simulink model "pidACCsystem"  (R2022a)
settings: Solver=FixedStepAuto  StartTime=0.0  StopTime=T  RelTol=1e-3
values from neighbouring files (symbols this model uses):
  t_gap = 1.4    [PreRun.m]
  Ts = 1e-2    (= 0.01)    [PreRun.m]
  v0_ego_1 = 20/9    (= 2.22222222222)    [PreRun.m]
  v0_ego_2 = 20/9    (= 2.22222222222)    [PreRun.m]
  v0_ego_3 = 20/9    (= 2.22222222222)    [PreRun.m]
  v0_lead = 25/9    (= 2.77777777778)    [PreRun.m]
  x0_ego_1 = x0_lead - (10 + t_gap*v0_ego_1)    (= 56.8888888889)    [PreRun.m]
  x0_ego_2 = x0_ego_1 - (10 + t_gap*v0_ego_2)    (= 43.7777777778)    [PreRun.m]
  x0_ego_3 = x0_ego_2 - (10 + t_gap*v0_ego_3)    (= 30.6666666667)    [PreRun.m]
  x0_lead = 70    [PreRun.m]
libraries: eeStairGenerator x1
settings Model: Creator=The MathWorks, Inc.  LastModifiedBy=SAMEER TALWAR
settings SolverCC: AlgebraicLoopSolver=TrustRegion
settings DataIOCC: ReturnWorkspaceOutputs=off
settings DebuggingCC: UnconnectedInputMsg=warning  UnconnectedOutputMsg=warning  UnconnectedLineMsg=warning  SFMachineParentedDataDiag=warning  ArithmeticOperatorsInVariantConditions=warning
settings SFSimCC: SimUseLocalCustomCode=off  CustomCodeUndefinedFunction=UseInterfaceOnly
settings RTWCC: RTWUseLocalCustomCode=off
settings CodeAppCC: StateflowObjectComments=on

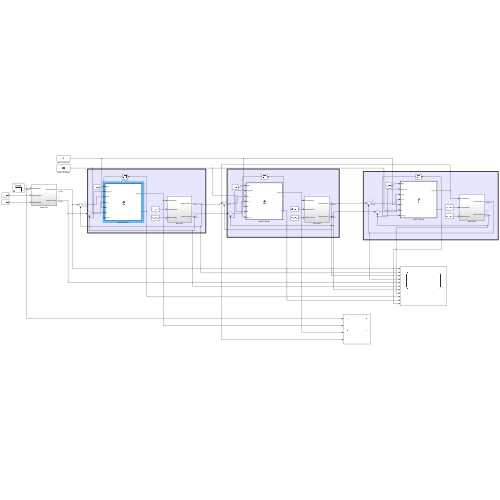
[thumbnail: Simulink's stored preview of the top-level diagram]
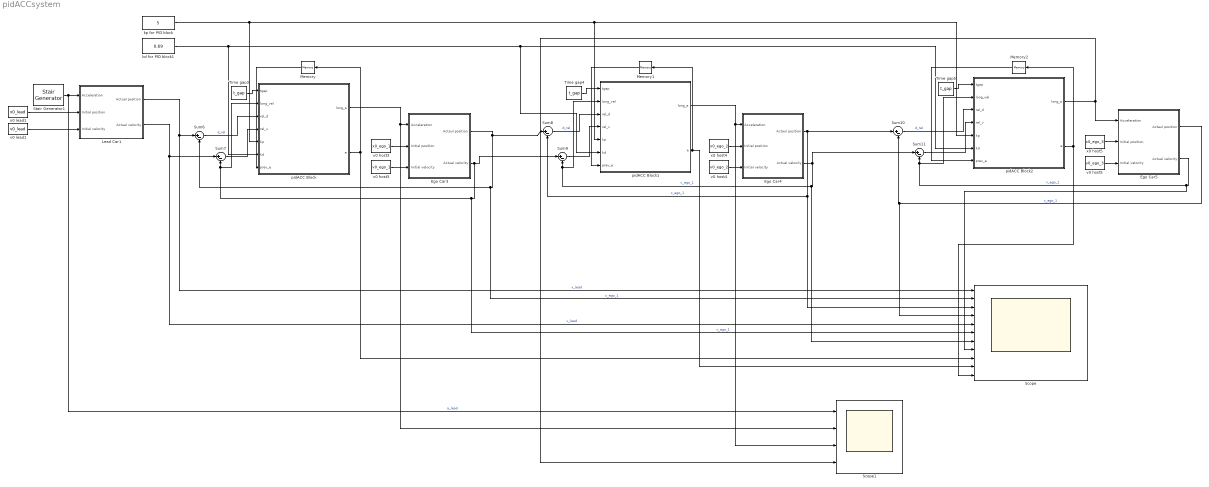
== system pidACCsystem ==
  Ego Car3 : Subsystem
  Ego Car4 : Subsystem
  Ego Car5 : Subsystem
  Lead Car1 : Subsystem
  Memory : Memory
  Memory1 : Memory
  Memory2 : Memory
  Scope : Scope  NumInputPorts=11
  Scope1 : Scope  NumInputPorts=4
  Stair Generator1 : eeStairGenerator/Stair Generator  LabelModeActiveChoice=Discrete  TimeInput=[35 37]  AmplitudeInput=[2 0 ]  SampleTime=Ts  RepeatPattern=off  OutDataTypeStr=double
      settings: SourceProductBaseCode=PS
  Sum{6..11} (6 alike) : Sum  Inputs=|+-
  Time gap3 : Constant  Value=t_gap  SampleTime=Ts
  Time gap4 : Constant  Value=t_gap  SampleTime=Ts
  Time gap5 : Constant  Value=t_gap  SampleTime=Ts
  kd for PID block1 : Constant  Value=0.69
  kp for PID block : Constant  Value=5
  pidACC Block : MATLAB Function  TreatAsAtomicUnit=on
  pidACC Block1 : MATLAB Function  TreatAsAtomicUnit=on
  pidACC Block2 : MATLAB Function  TreatAsAtomicUnit=on
  v0 host3 : Constant  Value=v0_ego_1  SampleTime=Ts
  v0 host4 : Constant  Value=v0_ego_2  SampleTime=Ts
  v0 host5 : Constant  Value=v0_ego_3  SampleTime=Ts
  v0 lead1 : Constant  Value=v0_lead  SampleTime=Ts
  x0 host3 : Constant  Value=x0_ego_1  SampleTime=Ts
  x0 host4 : Constant  Value=x0_ego_2  SampleTime=Ts
  x0 host5 : Constant  Value=x0_ego_3  SampleTime=Ts
  x0 lead1 : Constant  Value=x0_lead  SampleTime=Ts
  wires:
  x0 host3/1 -> Ego Car3/2(Initial position)
  v0 host3/1 -> Ego Car3/3(Initial velocity)
  x0 lead1/1 -> Lead Car1/2(Initial position)
  v0 lead1/1 -> Lead Car1/3(Initial velocity)
  v0 host4/1 -> Ego Car4/3(Initial velocity)
  x0 host4/1 -> Ego Car4/2(Initial position)
  pidACC Block1/1(long_a) -> Scope1/3, Ego Car4/1(Acceleration)
  pidACC Block/1(long_a) -> Scope1/2, Ego Car3/1(Acceleration)
  x0 host5/1 -> Ego Car5/2(Initial position)
  v0 host5/1 -> Ego Car5/3(Initial velocity)
  pidACC Block2/1(long_a) -> Ego Car5/1(Acceleration), Scope1/4
  Stair Generator1/1 -> Scope1/1, Lead Car1/1(Acceleration)  "a_lead"
  Sum6/1 -> pidACC Block/3(rel_d)  "d_rel"
  Sum7/1 -> pidACC Block/4(rel_v)
  Ego Car3/2(Actual velocity) -> Sum9/1, Scope/6, pidACC Block/2(long_vel), Sum7/2  "v_ego_1"
  Lead Car1/2(Actual velocity) -> Scope/5, Sum7/1  "v_lead"
  Lead Car1/1(Actual position) -> Scope/1, Sum6/1  "x_lead"
  Ego Car3/1(Actaul position) -> Sum8/1, Scope/2, Sum6/2  "x_ego_1"
  Sum8/1 -> pidACC Block1/3(rel_d)  "d_rel"
  Sum9/1 -> pidACC Block1/4(rel_v)
  Ego Car4/2(Actual velocity) -> Scope/7, pidACC Block1/2(long_vel), Sum9/2, Sum11/1  "v_ego_1"
  Ego Car4/1(Actaul position) -> Scope/3, Sum8/2, Sum10/1  "x_ego_1"
  Sum10/1 -> pidACC Block2/3(rel_d)  "d_rel"
  Sum11/1 -> pidACC Block2/4(rel_v)
  Ego Car5/2(Actual velocity) -> Scope/8, pidACC Block2/2(long_vel), Sum11/2  "v_ego_1"
  Ego Car5/1(Actaul position) -> Scope/4, Sum10/2  "x_ego_1"
  Time gap3/1 -> pidACC Block/1(tgap)
  Time gap4/1 -> pidACC Block1/1(tgap)
  Time gap5/1 -> pidACC Block2/1(tgap)
  pidACC Block/2(e) -> Memory/1, Scope/9
  pidACC Block1/2(e) -> Memory1/1, Scope/10
  pidACC Block2/2(e) -> Memory2/1, Scope/11
  kp for PID block/1 -> pidACC Block2/5(kp), pidACC Block1/5(kp), pidACC Block/5(kp)
  Memory/1 -> pidACC Block/7(prev_e)
  kd for PID block1/1 -> pidACC Block1/6(kd), pidACC Block2/6(kd), pidACC Block/6(kd)
  Memory1/1 -> pidACC Block1/7(prev_e)
  Memory2/1 -> pidACC Block2/7(prev_e)

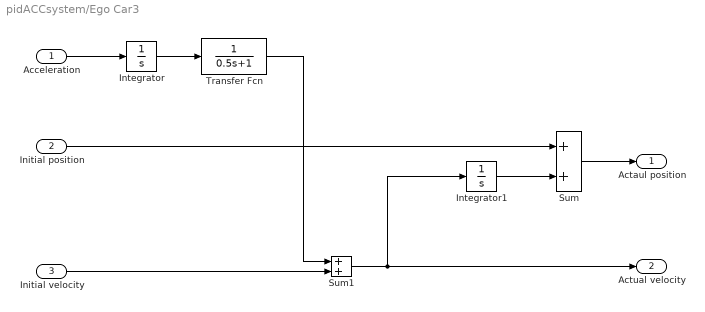
== system pidACCsystem/Ego Car3 ==
  Acceleration : Inport
  Initial position : Inport  Port=2
  Initial velocity : Inport  Port=3
  Integrator : Integrator
  Integrator1 : Integrator
  Sum : Sum
  Sum1 : Sum
  Transfer Fcn : TransferFcn  Denominator=[0.5 1]
  Actaul position : Outport  VectorParamsAs1DForOutWhenUnconnected=off
  Actual velocity : Outport  Port=2  VectorParamsAs1DForOutWhenUnconnected=off
  wires:
  Sum1/1 -> Integrator1/1, Actual velocity/1
  Initial velocity/1 -> Sum1/2
  Sum/1 -> Actaul position/1
  Transfer Fcn/1 -> Sum1/1
  Integrator/1 -> Transfer Fcn/1
  Acceleration/1 -> Integrator/1
  Initial position/1 -> Sum/1
  Integrator1/1 -> Sum/2

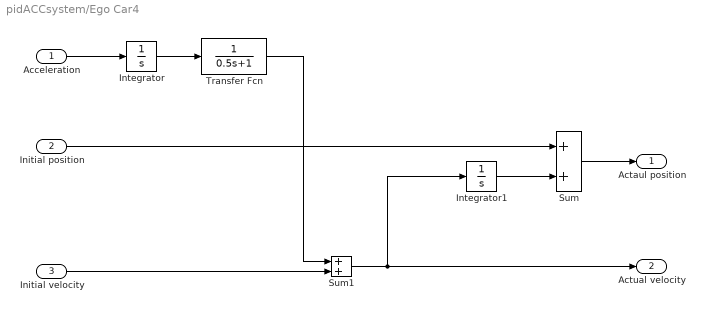
== system pidACCsystem/Ego Car4 ==
  Acceleration : Inport
  Initial position : Inport  Port=2
  Initial velocity : Inport  Port=3
  Integrator : Integrator
  Integrator1 : Integrator
  Sum : Sum
  Sum1 : Sum
  Transfer Fcn : TransferFcn  Denominator=[0.5 1]
  Actaul position : Outport  VectorParamsAs1DForOutWhenUnconnected=off
  Actual velocity : Outport  Port=2  VectorParamsAs1DForOutWhenUnconnected=off
  wires:
  Sum1/1 -> Integrator1/1, Actual velocity/1
  Initial velocity/1 -> Sum1/2
  Sum/1 -> Actaul position/1
  Transfer Fcn/1 -> Sum1/1
  Integrator/1 -> Transfer Fcn/1
  Acceleration/1 -> Integrator/1
  Initial position/1 -> Sum/1
  Integrator1/1 -> Sum/2

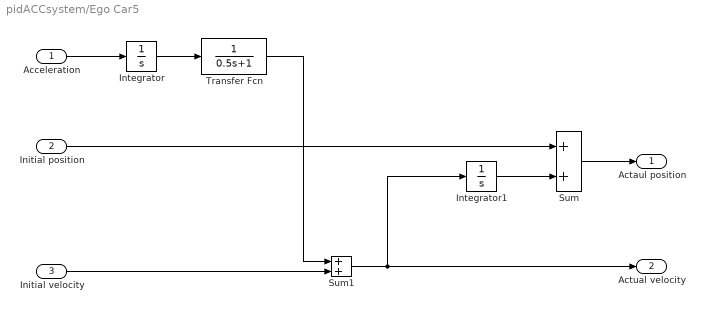
== system pidACCsystem/Ego Car5 ==
  Acceleration : Inport
  Initial position : Inport  Port=2
  Initial velocity : Inport  Port=3
  Integrator : Integrator
  Integrator1 : Integrator
  Sum : Sum
  Sum1 : Sum
  Transfer Fcn : TransferFcn  Denominator=[0.5 1]
  Actaul position : Outport  VectorParamsAs1DForOutWhenUnconnected=off
  Actual velocity : Outport  Port=2  VectorParamsAs1DForOutWhenUnconnected=off
  wires:
  Sum1/1 -> Integrator1/1, Actual velocity/1
  Initial velocity/1 -> Sum1/2
  Sum/1 -> Actaul position/1
  Transfer Fcn/1 -> Sum1/1
  Integrator/1 -> Transfer Fcn/1
  Acceleration/1 -> Integrator/1
  Initial position/1 -> Sum/1
  Integrator1/1 -> Sum/2

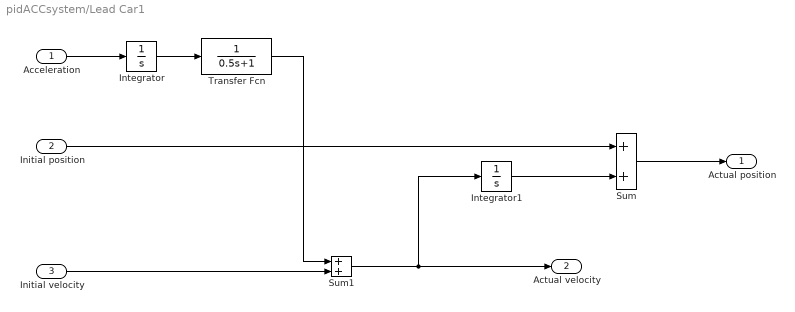
== system pidACCsystem/Lead Car1 ==
  Acceleration : Inport
  Initial position : Inport  Port=2
  Initial velocity : Inport  Port=3
  Integrator : Integrator
  Integrator1 : Integrator
  Sum : Sum
  Sum1 : Sum
  Transfer Fcn : TransferFcn  Denominator=[0.5 1]
  Actual position : Outport  VectorParamsAs1DForOutWhenUnconnected=off
  Actual velocity : Outport  Port=2  VectorParamsAs1DForOutWhenUnconnected=off
  wires:
  Integrator1/1 -> Sum/2
  Initial position/1 -> Sum/1
  Acceleration/1 -> Integrator/1
  Sum1/1 -> Actual velocity/1, Integrator1/1
  Integrator/1 -> Transfer Fcn/1
  Sum/1 -> Actual position/1
  Initial velocity/1 -> Sum1/2
  Transfer Fcn/1 -> Sum1/1

== matlab function pidACCsystem/pidACC Block ==
  data: tgap input; long_a output; long_vel input; rel_d input; rel_v input; e output; kp input; kd input; prev_e input
function [long_a,e] = fcn(tgap, long_vel, rel_d, rel_v, kp, kd, prev_e)
dt=0.01;
dsafe = 10 + (tgap*long_vel);
e = rel_d - dsafe;
long_a = kp*e + kd*(e-prev_e)/dt;

== matlab function pidACCsystem/pidACC Block1 ==
  data: tgap input; long_a output; long_vel input; rel_d input; rel_v input; e output; kp input; kd input; prev_e input
function [long_a,e] = fcn(tgap, long_vel, rel_d, rel_v, kp, kd, prev_e)
dt=0.01;
dsafe = 10 + (tgap*long_vel);
e = rel_d - dsafe;
long_a = kp*e + kd*(e-prev_e)/dt;

== matlab function pidACCsystem/pidACC Block2 ==
  data: tgap input; long_a output; long_vel input; rel_d input; rel_v input; e output; kp input; kd input; prev_e input
function [long_a,e] = fcn(tgap, long_vel, rel_d, rel_v, kp, kd, prev_e)
dt=0.01;
dsafe = 10 + (tgap*long_vel);
e = rel_d - dsafe;
long_a = kp*e + kd*(e-prev_e)/dt;
